simulink model "LQGIArduino"  (R2019b)
settings: Solver=FixedStepAuto  StartTime=0.0  StopTime=Inf  RelTol=1e-3  EnableMultiTasking=on
values from neighbouring files (symbols this model uses):
  h0 = geometry_parameters(3)    [CalculateLoadCapacity.m]    (also in initialiseradialgap.m; main.m = 5e-05)
  Klqgi = lqr(Aaug,Baug,Qaug,Raug)    [main.m]
  syskfd = c2d(syskf,Ts)    [main.m]
  Ts = 1/fs    (= 0.001)    [main.m]
undefined symbols (not defined in the file or in its folder): DiscIntNeverNeededParam
libraries: arduinolib x2
settings Model: SILPILModeSetting=veronly  ExtModeTrigDuration=2  Creator=Alexander  LastModifiedBy=Alexander
settings SolverCC: AutoInsertRateTranBlk=on
settings OptimizationCC: EnhancedBackFolding=on  PassReuseOutputArgsAs=Individual arguments  ZeroExternalMemoryAtStartup=off  ZeroInternalMemoryAtStartup=off  MaxStackSize=64  OptimizeBlockOrder=speed  DifferentSizesBufferReuse=on  OptimizationCustomize=off  EfficientTunableParamExpr=on
settings DebuggingCC: ParameterTunabilityLossMsg=error
settings HardwareCC: ProdBitPerInt=16  ProdBitPerPointer=16  ProdBitPerSizeT=16  ProdBitPerPtrDiffT=16  ProdLargestAtomicFloat=None  ProdWordSize=8  ProdHWDeviceType=Atmel->AVR
settings SFSimCC: MATLABDynamicMemAlloc=off
settings RTWCC: SystemTargetFile=ert.tlc  HardwareBoard=Arduino Mega 2560  TLCOptions=-aInlineSetEventsForThisBaseRateFcn=TLC_FALSE -aSuppressMultiTaskScheduler=TLC_FALSE -aRateBasedStepFcn=1  TemplateMakefile=ert_default_tmf  GenerateReport=on  Toolchain=Arduino AVR  BuildConfiguration=Faster Runs  IncludeHyperlinkInReport=on  LaunchReport=on  GenerateTraceInfo=on  GenerateTraceReport=on  GenerateTraceReportSl=on  GenerateTraceReportSf=on  GenerateTraceReportEml=on
settings CodeAppCC: ForceParamTrailComments=on  IgnoreCustomStorageClasses=off  OperatorAnnotations=on  SimulinkDataObjDesc=on  SFDataObjDesc=on  InsertBlockDesc=on
settings ERTTargetCC: SupportContinuousTime=on  SupportVariableSizeSignals=on  ExtModeStaticAllocSize=2048

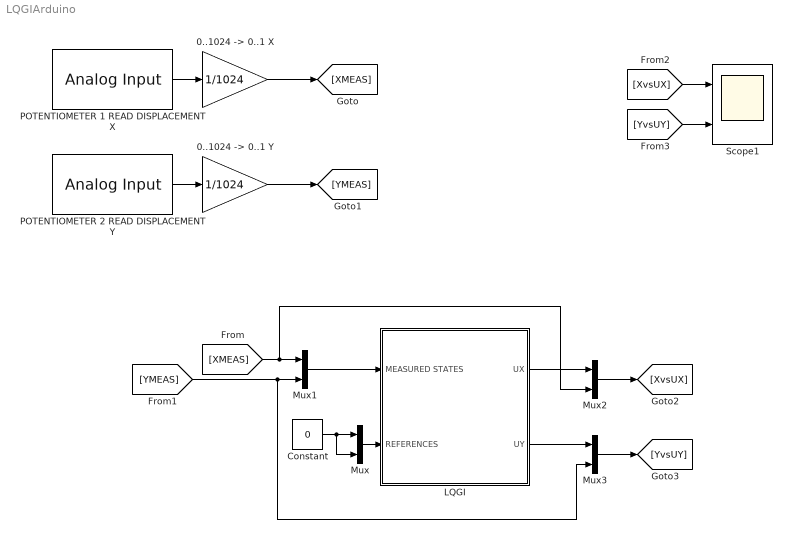
== system LQGIArduino ==
  "0..1024 -> 0..1 X" : Gain  Gain=1/1024  OutDataTypeStr=double
  "0..1024 -> 0..1 Y" : Gain  Gain=1/1024  OutDataTypeStr=double
  Constant : Constant  Value=0
  LQGI : Subsystem
  Mux{,1..3} (4 alike) : Mux  Inputs=2
  POTENTIOMETER 1 READ DISPLACEMENT X : arduinolib/Analog Input  pinNumber=0  ReadResultsOnly=off  ConversionTriggerSource=Software  ExternalTriggerType=uint32(0)  OutputDataType=uint16  EnableConversionCompleteNotify=off  EnableOuputStatus=off  SampleTime=0.001  blockPlatform=arduino
  POTENTIOMETER 2 READ DISPLACEMENT Y : arduinolib/Analog Input  pinNumber=1  ReadResultsOnly=off  ConversionTriggerSource=Software  ExternalTriggerType=uint32(0)  OutputDataType=uint16  EnableConversionCompleteNotify=off  EnableOuputStatus=off  SampleTime=0.001  blockPlatform=arduino
  Scope1 : Scope  NumInputPorts=2
  wires:
  Mux/1 -> LQGI/2(REFERENCES)
  Constant/1 -> Mux/2, Mux/1
  POTENTIOMETER 2 READ DISPLACEMENT Y/1 -> "0..1024 -> 0..1 Y"/1
  POTENTIOMETER 1 READ DISPLACEMENT X/1 -> "0..1024 -> 0..1 X"/1
  Mux1/1 -> LQGI/1(MEASURED STATES)
  LQGI/1(UX) -> Mux2/1
  LQGI/2("UY ") -> Mux3/1
  "0..1024 -> 0..1 X"/1 -> [XMEAS]
  "0..1024 -> 0..1 Y"/1 -> [YMEAS]
  [XMEAS] -> Mux2/2, Mux1/1
  [YMEAS] -> Mux3/2, Mux1/2
  Mux2/1 -> [XvsUX]
  Mux3/1 -> [YvsUY]
  [XvsUX] -> Scope1/1
  [YvsUY] -> Scope1/2

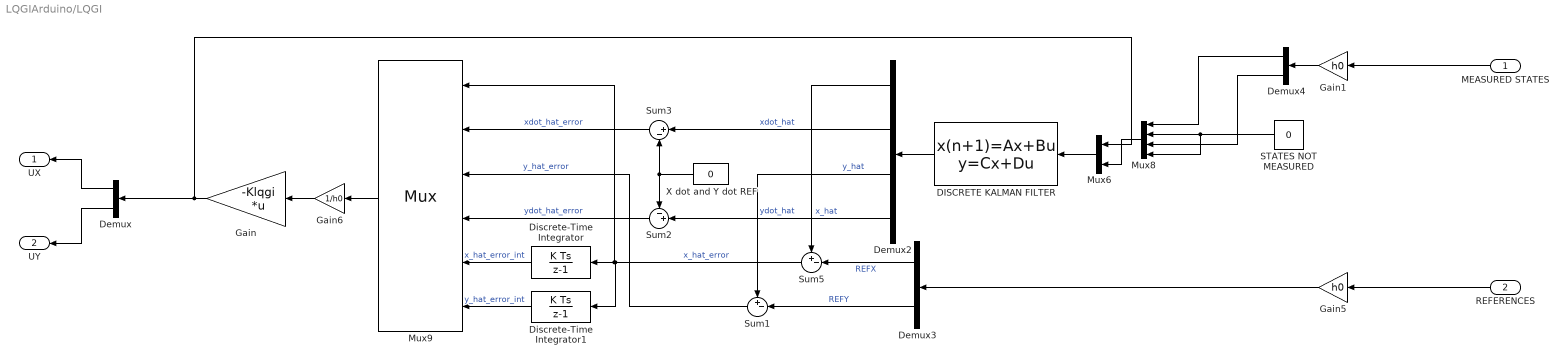
== system LQGIArduino/LQGI ==
  MEASURED STATES : Inport  OutDataTypeStr=double
  REFERENCES : Inport  Port=2  OutDataTypeStr=double
  DISCRETE KALMAN FILTER : DiscreteStateSpace  A=syskfd.A  B=syskfd.B  C=syskfd.C  D=syskfd.D  SampleTime=Ts
  Demux : Demux  Outputs=2
  Demux2 : Demux
  Demux3 : Demux  Outputs=2
  Demux4 : Demux  Outputs=2
  Discrete-Time Integrator : DiscreteIntegrator  SampleTime=Ts  LimitOutput=on  UpperSaturationLimit=1e-5  LowerSaturationLimit=-1e-5  IgnoreLimit=on  ICPrevOutput=DiscIntNeverNeededParam  ICPrevScaledInput=DiscIntNeverNeededParam
  Discrete-Time Integrator1 : DiscreteIntegrator  SampleTime=Ts  LimitOutput=on  UpperSaturationLimit=1e-5  LowerSaturationLimit=-1e-5  IgnoreLimit=on  ICPrevOutput=DiscIntNeverNeededParam  ICPrevScaledInput=DiscIntNeverNeededParam
  Gain : Gain  Gain=-Klqgi  Multiplication=Matrix(K*u) (u vector)
  Gain1 : Gain  Gain=h0
  Gain5 : Gain  Gain=h0
  Gain6 : Gain  Gain=1/h0
  Mux6 : Mux  Inputs=2
  Mux8 : Mux
  Mux9 : Mux  Inputs=6
      settings: DisplayOption=signals
  STATES NOT MEASURED : Constant  Value=0
  Sum1 : Sum  Inputs=+-|
  Sum2 : Sum  Inputs=-+|
  Sum3 : Sum  Inputs=|+-
  Sum5 : Sum  Inputs=+-|
  X dot and Y dot REF : Constant  Value=0
  UX : Outport  OutDataTypeStr=double
  "UY " : Outport  Port=2  OutDataTypeStr=double
  wires:
  Demux2/1 -> Sum5/1  "x_hat"
  Gain6/1 -> Gain/1
  Mux6/1 -> DISCRETE KALMAN FILTER/1
  Demux4/1 -> Mux8/1
  DISCRETE KALMAN FILTER/1 -> Demux2/1
  Demux3/1 -> Sum5/2  "REFX"
  Gain1/1 -> Demux4/1
  Gain/1 -> Mux6/1, Demux/1
  Mux9/1 -> Gain6/1
  Sum1/1 -> Mux9/3  "y_hat_error"
  MEASURED STATES/1 -> Gain1/1
  Mux8/1 -> Mux6/2
  STATES NOT MEASURED/1 -> Mux8/4, Mux8/2
  Demux4/2 -> Mux8/3
  Sum3/1 -> Mux9/2  "xdot_hat_error"
  Demux/1 -> UX/1
  Sum5/1 -> Discrete-Time Integrator1/1, Discrete-Time Integrator/1, Mux9/1  "x_hat_error"
  Demux2/2 -> Sum3/1  "xdot_hat"
  X dot and Y dot REF/1 -> Sum2/1, Sum3/2
  Demux3/2 -> Sum1/2  "REFY"
  Sum2/1 -> Mux9/4  "ydot_hat_error"
  Demux2/3 -> Sum1/1  "y_hat"
  Demux2/4 -> Sum2/2  "ydot_hat"
  Gain5/1 -> Demux3/1
  Demux/2 -> "UY "/1
  REFERENCES/1 -> Gain5/1
  Discrete-Time Integrator/1 -> Mux9/5  "x_hat_error_int"
  Discrete-Time Integrator1/1 -> Mux9/6  "y_hat_error_int"
